simulink model "CopterSim3DEnvironment"  (R2019b)
settings: Solver=ode4  StartTime=0.0  StopTime=inf  FixedStep=0.001  RelTol=1e-3
InitFcn:
  | Init_control;
values from neighbouring files (symbols this model uses):
  Kd_RP_AgngleRate = 0.005    [Init_control.m]    (also in quadFly.sldd)
  Kd_YAW_AngleRate = 0.05    [Init_control.m]    (also in quadFly.sldd)
  Ki_RP_AgngleRate = 0.01    [Init_control.m]    (also in quadFly.sldd)
  Ki_YAW_AngleRate = 0.8    [Init_control.m]    (also in quadFly.sldd)
  Kp_RP_AgngleRate = 0.55    [Init_control.m]    (also in quadFly.sldd)
  Kp_RP_ANGLE = 6.5    [Init_control.m]    (also in quadFly.sldd)
  Kp_YAW_AngleRate = 3.2    [Init_control.m]    (also in quadFly.sldd)
  MAX_CONTROL_ANGLE_RATE_Y = 90    [Init_control.m]    (also in quadFly.sldd = 90.0)
  ModelInit_RPM = 0.0    [quadFly.sldd]
  ModelParam_envAltitude = -41.5260009765625    [quadFly.sldd]
  ModelParam_GlobalNoiseGainSwitch = 1.0    [quadFly.sldd]
  ModelParam_GPSLatLong = 40.1540302 116.2593683    [quadFly.sldd]
  ModelParam_motorCr = 1148.0    [quadFly.sldd]
  ModelParam_motorJm = 0.0001287    [quadFly.sldd]
  ModelParam_motorMinThr = 0.05    [quadFly.sldd]
  ModelParam_motorT = 0.02    [quadFly.sldd]
  ModelParam_motorWb = -141.4    [quadFly.sldd]
  ModelParam_rotorCm = 1.779E-7    [quadFly.sldd]
  ModelParam_rotorCt = 1.105E-5    [quadFly.sldd]
  ModelParam_uavCCm = 0.01 0.01 0.0055    [quadFly.sldd]
  ModelParam_uavCd = 0.073    [quadFly.sldd]
  ModelParam_uavDearo = 0.12    [quadFly.sldd]
  ModelParam_uavJ = 0.0211 0.0 0.0 0.0 0.0219 0.0 0.0 0.0 0.0366    [quadFly.sldd]
  ModelParam_uavMass = 1.4    [quadFly.sldd]
  ModelParam_uavR = 0.225    [quadFly.sldd]
  ModelParam_uavType = 3    [quadFly.sldd]
undefined symbols (not defined in the file or in its folder): DWORK0, DWORK1, DWORK10, DWORK11, DWORK12, DWORK13, DWORK14, DWORK15, DWORK2, DWORK3, DWORK4, DWORK5, DWORK6, DWORK7, DWORK8, DWORK9, earthRadius, KiPitchAttitude, KiRollAttitude, Receive, Send
libraries: simulink x15, ctrl_ADRC_angular_rate x4, aerolibfltsims x3, ctrl_ADRC_TD x2, shared6dof x1, aerolibanimutils x1
(part 3 of 4)

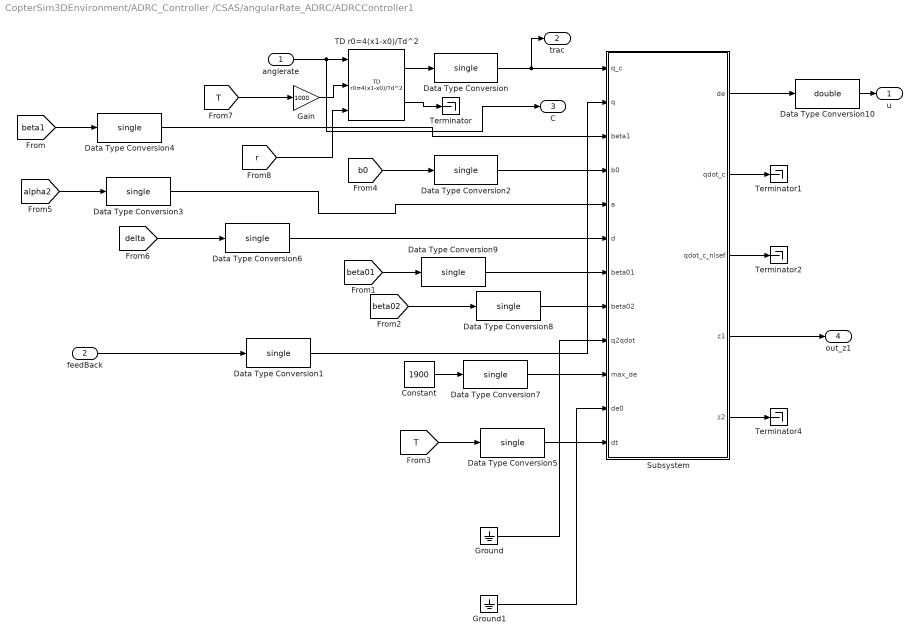
== system CopterSim3DEnvironment/ADRC_Controller /CSAS/angularRate_ADRC/ADRCController1 ==
  anglerate : Inport
  feedBack : Inport  Port=2
  Constant : Constant  Value=1900
  Data Type Conversion{,1..9} (10 alike) : DataTypeConversion  OutDataTypeStr=single
  Data Type Conversion10 : DataTypeConversion  OutDataTypeStr=double
  Gain : Gain  Gain=1000
  Ground : Ground
  Ground1 : Ground
  Subsystem : Subsystem  AncestorBlock=ctrl_ADRC_angular_rate/Subsystem  mask(ADRC angular rate controller){}
      mask help: 二阶ADRC姿态角速率控制
  TD r0=4(x1-x0)/Td^2 : ctrl_ADRC_TD/TD r0=4(x1-x0)//Td^2
  Terminator{,1..2,4} (4 alike) : Terminator
  u : Outport
  trac : Outport  Port=2
  C : Outport  Port=3
  out_z1 : Outport  Port=4
  wires:
  Constant/1 -> Data Type Conversion7/1
  Ground/1 -> Subsystem/9(q2qdot)
  Data Type Conversion1/1 -> Subsystem/2(q)
  Data Type Conversion/1 -> trac/1, Subsystem/1(q_c)
  [beta01] -> Data Type Conversion9/1
  [delta] -> Data Type Conversion6/1
  [r] -> TD r0=4(x1-x0)/Td^2/3
  [beta1] -> Data Type Conversion4/1
  [alpha2] -> Data Type Conversion3/1
  [T] -> Gain/1
  Ground1/1 -> Subsystem/11(de0)
  feedBack/1 -> Data Type Conversion1/1
  [b0] -> Data Type Conversion2/1
  [T] -> Data Type Conversion5/1
  [beta02] -> Data Type Conversion8/1
  Subsystem/5(z2) -> Terminator4/1
  Subsystem/4(z1) -> out_z1/1
  Subsystem/2(qdot_c) -> Terminator1/1
  Subsystem/3(qdot_c_nlsef) -> Terminator2/1
  anglerate/1 -> C/1, TD r0=4(x1-x0)/Td^2/1
  Subsystem/1(de) -> Data Type Conversion10/1
  TD r0=4(x1-x0)/Td^2/2 -> Terminator/1
  TD r0=4(x1-x0)/Td^2/1 -> Data Type Conversion/1
  Data Type Conversion2/1 -> Subsystem/4(b0)
  Data Type Conversion4/1 -> Subsystem/3(beta1)
  Data Type Conversion3/1 -> Subsystem/5(a)
  Data Type Conversion6/1 -> Subsystem/6(d)
  Data Type Conversion5/1 -> Subsystem/12(dt)
  Data Type Conversion7/1 -> Subsystem/10(max_de)
  Data Type Conversion8/1 -> Subsystem/8(beta02)
  Data Type Conversion9/1 -> Subsystem/7(beta01)
  Data Type Conversion10/1 -> u/1
  Gain/1 -> TD r0=4(x1-x0)/Td^2/2

== system CopterSim3DEnvironment/ADRC_Controller /CSAS/angularRate_ADRC/ADRCController2 ==
  anglerate : Inport
  angleRateBack : Inport  Port=2
  Add : Sum  Inputs=+-
  Add1 : Sum  Inputs=+-
  Add2 : Sum  Inputs=+-
  Divide : Product  Inputs=*/
  NLSEF : Subsystem
  TD : Subsystem
  Unit Delay : UnitDelay  SampleTime=-1  HasFrameUpgradeWarning=on
  eso : Subsystem
  u : Outport
  wires:
  anglerate/1 -> TD/1(anglerate)
  TD/1(anglerateV1) -> Add/1
  TD/2(angleAccV2) -> Add1/1
  eso/1(z1) -> Add/2
  eso/2(z2) -> Add1/2
  Add/1 -> NLSEF/1(e1)
  Add1/1 -> NLSEF/2(e2)
  eso/3(z3) -> Add2/2
  NLSEF/1(u0) -> Add2/1
  Add2/1 -> Unit Delay/1, Divide/1
  [b0] -> Divide/2
  Divide/1 -> u/1
  angleRateBack/1 -> eso/1(phi_rate)
  Unit Delay/1 -> eso/2(angle_u)

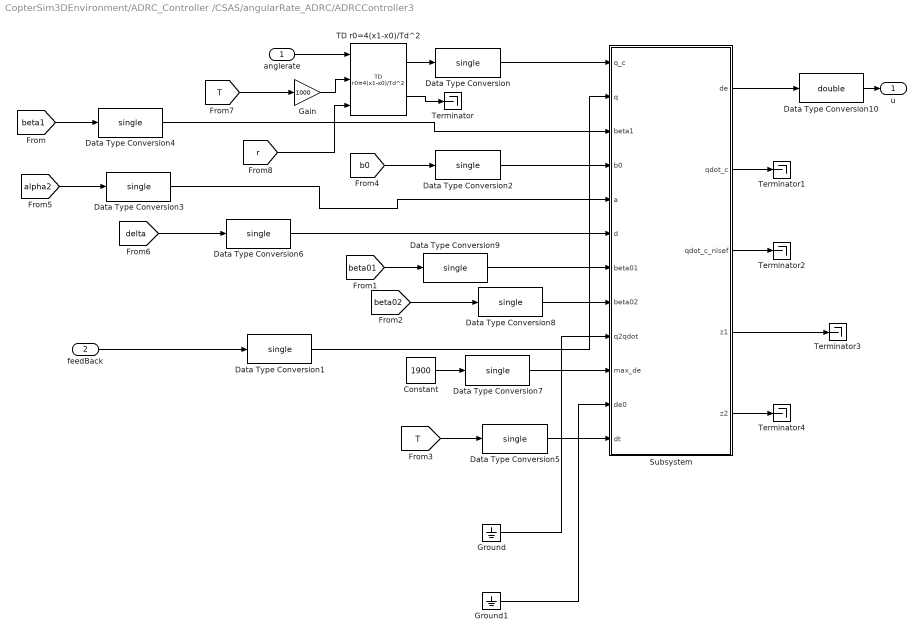
== system CopterSim3DEnvironment/ADRC_Controller /CSAS/angularRate_ADRC/ADRCController3 ==
  anglerate : Inport
  feedBack : Inport  Port=2
  Constant : Constant  Value=1900
  Data Type Conversion{,1..9} (10 alike) : DataTypeConversion  OutDataTypeStr=single
  Data Type Conversion10 : DataTypeConversion  OutDataTypeStr=double
  Gain : Gain  Gain=1000
  Ground : Ground
  Ground1 : Ground
  Subsystem : Subsystem  AncestorBlock=ctrl_ADRC_angular_rate/Subsystem  mask(ADRC angular rate controller){}
      mask help: 二阶ADRC姿态角速率控制
  TD r0=4(x1-x0)/Td^2 : ctrl_ADRC_TD/TD r0=4(x1-x0)//Td^2
  Terminator{,1..4} (5 alike) : Terminator
  u : Outport
  wires:
  Constant/1 -> Data Type Conversion7/1
  Ground/1 -> Subsystem/9(q2qdot)
  Data Type Conversion1/1 -> Subsystem/2(q)
  Data Type Conversion/1 -> Subsystem/1(q_c)
  [beta01] -> Data Type Conversion9/1
  [delta] -> Data Type Conversion6/1
  [r] -> TD r0=4(x1-x0)/Td^2/3
  [beta1] -> Data Type Conversion4/1
  [alpha2] -> Data Type Conversion3/1
  [T] -> Gain/1
  Ground1/1 -> Subsystem/11(de0)
  feedBack/1 -> Data Type Conversion1/1
  [b0] -> Data Type Conversion2/1
  [T] -> Data Type Conversion5/1
  [beta02] -> Data Type Conversion8/1
  Subsystem/5(z2) -> Terminator4/1
  Subsystem/4(z1) -> Terminator3/1
  Subsystem/2(qdot_c) -> Terminator1/1
  Subsystem/3(qdot_c_nlsef) -> Terminator2/1
  anglerate/1 -> TD r0=4(x1-x0)/Td^2/1
  Subsystem/1(de) -> Data Type Conversion10/1
  TD r0=4(x1-x0)/Td^2/2 -> Terminator/1
  TD r0=4(x1-x0)/Td^2/1 -> Data Type Conversion/1
  Data Type Conversion2/1 -> Subsystem/4(b0)
  Data Type Conversion4/1 -> Subsystem/3(beta1)
  Data Type Conversion3/1 -> Subsystem/5(a)
  Data Type Conversion6/1 -> Subsystem/6(d)
  Data Type Conversion5/1 -> Subsystem/12(dt)
  Data Type Conversion7/1 -> Subsystem/10(max_de)
  Data Type Conversion8/1 -> Subsystem/8(beta02)
  Data Type Conversion9/1 -> Subsystem/7(beta01)
  Data Type Conversion10/1 -> u/1
  Gain/1 -> TD r0=4(x1-x0)/Td^2/2

== system CopterSim3DEnvironment/ADRC_Controller /CSAS/angularRate_ADRC/Subsystem ==
  yaw : Inport
  q : Inport  Port=2
  r : Inport  Port=3
  pitchRateCom : Inport  Port=4
  Sum17 : Sum  Inputs=|-+
  Sum21 : Sum  Inputs=|-+
  pitch_rate : simulink/Continuous/PID Controller  Controller=PID  Form=Parallel  TimeDomain=Discrete-time  SampleTime=-1  IntegratorMethod=Forward Euler  FilterMethod=Forward Euler  ControllerParametersSource=internal  P=Kp_RP_AgngleRate  I=Ki_RP_AgngleRate  D=Kd_RP_AgngleRate  UseFilter=off  N=100  TunerSelectOption=Transfer Function Based (PID Tuner App)  InitialConditionSource=internal  InitialConditionForIntegrator=0  InitialConditionForFilter=0  DifferentiatorICPrevScaledInput=0  ExternalReset=none  TrackingMode=off  Kt=1  LimitOutput=on  UpperSaturationLimit=500  LowerSaturationLimit=-500  LinearizeAsGain=on  AntiWindupMode=back-calculation  Kb=1  POutMin=[]  POutMax=[]  IOutMin=[]  IOutMax=[]  DOutMin=[]  DOutMax=[]  NOutMin=[]  NOutMax=[]  SumOutMin=[]  SumOutMax=[]  SaturationOutMin=[]  SaturationOutMax=[]  PParamMin=[]  PParamMax=[]  IParamMin=[]  IParamMax=[]  DParamMin=[]  DParamMax=[]  NParamMin=[]  NParamMax=[]  KbParamMin=[]  KbParamMax=[]  KtParamMin=[]  KtParamMax=[]  KbOutMin=[]  KbOutMax=[]  KtOutMin=[]  KtOutMax=[]  IntegratorOutMin=[]  IntegratorOutMax=[]  FilterOutMin=[]  FilterOutMax=[]  SumI1OutMin=[]  SumI1OutMax=[]  SumI2OutMin=[]  SumI2OutMax=[]  SumI3OutMin=[]  SumI3OutMax=[]  SumI4OutMin=[]  SumI4OutMax=[]  SumDOutMin=[]  SumDOutMax=[]  DifferentiatorOutMin=[]  DifferentiatorOutMax=[]  FilterDiffOutCoefMin=[]  FilterDiffOutCoefMax=[]  ReciprocalOutMin=[]  ReciprocalOutMax=[]  SumDenOutMin=[]  SumDenOutMax=[]  SumNumOutMin=[]  SumNumOutMax=[]  DivideOutMin=[]  DivideOutMax=[]  IntegratorContinuousStateAttributes=''  IntegratorStateMustResolveToSignalObject=off  IntegratorRTWStateStorageClass=Auto  FilterContinuousStateAttributes=''  FilterStateMustResolveToSignalObject=off  FilterRTWStateStorageClass=Auto  ParallelPVariant=InternalParameters  IdealPVariant=Disabled  IVariant=InternalParameters  DVariant=InternalParameters  IntegratorVariant=Discrete  SatVariant=Enabled  AWVariant=BackCalculation  PCopyVariant=Disabled  TRVariant=Disabled  FdbkBlocksVariant=Forward  IdealPFdbkVariant=Disabled  SatFdbkVariant=Disabled  DerivativeFilterVariant=Differentiator  NVariant=Passthrough  NCopyVariant=Disabled_SignalSpec  FilterICVariant=InternalICsDifferentiator  IntegratorICVariant=InternalICs  ExternalResetVariant=Disabled  TRSumVariant=Passthrough  SumFdbkVariant=Disabled  SumVariant=Sum_PID
  yaw_rate : simulink/Continuous/PID Controller  Controller=PID  Form=Parallel  TimeDomain=Discrete-time  SampleTime=-1  IntegratorMethod=Forward Euler  FilterMethod=Forward Euler  ControllerParametersSource=internal  P=Kp_YAW_AngleRate  I=Ki_YAW_AngleRate  D=Kd_YAW_AngleRate  UseFilter=off  N=100  TunerSelectOption=Transfer Function Based (PID Tuner App)  InitialConditionSource=internal  InitialConditionForIntegrator=0  InitialConditionForFilter=0  DifferentiatorICPrevScaledInput=0  ExternalReset=none  TrackingMode=off  Kt=1  LimitOutput=on  UpperSaturationLimit=500  LowerSaturationLimit=-500  LinearizeAsGain=on  AntiWindupMode=back-calculation  Kb=1  POutMin=[]  POutMax=[]  IOutMin=[]  IOutMax=[]  DOutMin=[]  DOutMax=[]  NOutMin=[]  NOutMax=[]  SumOutMin=[]  SumOutMax=[]  SaturationOutMin=[]  SaturationOutMax=[]  PParamMin=[]  PParamMax=[]  IParamMin=[]  IParamMax=[]  DParamMin=[]  DParamMax=[]  NParamMin=[]  NParamMax=[]  KbParamMin=[]  KbParamMax=[]  KtParamMin=[]  KtParamMax=[]  KbOutMin=[]  KbOutMax=[]  KtOutMin=[]  KtOutMax=[]  IntegratorOutMin=[]  IntegratorOutMax=[]  FilterOutMin=[]  FilterOutMax=[]  SumI1OutMin=[]  SumI1OutMax=[]  SumI2OutMin=[]  SumI2OutMax=[]  SumI3OutMin=[]  SumI3OutMax=[]  SumI4OutMin=[]  SumI4OutMax=[]  SumDOutMin=[]  SumDOutMax=[]  DifferentiatorOutMin=[]  DifferentiatorOutMax=[]  FilterDiffOutCoefMin=[]  FilterDiffOutCoefMax=[]  ReciprocalOutMin=[]  ReciprocalOutMax=[]  SumDenOutMin=[]  SumDenOutMax=[]  SumNumOutMin=[]  SumNumOutMax=[]  DivideOutMin=[]  DivideOutMax=[]  IntegratorContinuousStateAttributes=''  IntegratorStateMustResolveToSignalObject=off  IntegratorRTWStateStorageClass=Auto  FilterContinuousStateAttributes=''  FilterStateMustResolveToSignalObject=off  FilterRTWStateStorageClass=Auto  ParallelPVariant=InternalParameters  IdealPVariant=Disabled  IVariant=InternalParameters  DVariant=InternalParameters  IntegratorVariant=Discrete  SatVariant=Enabled  AWVariant=BackCalculation  PCopyVariant=Disabled  TRVariant=Disabled  FdbkBlocksVariant=Forward  IdealPFdbkVariant=Disabled  SatFdbkVariant=Disabled  DerivativeFilterVariant=Differentiator  NVariant=Passthrough  NCopyVariant=Disabled_SignalSpec  FilterICVariant=InternalICsDifferentiator  IntegratorICVariant=InternalICs  ExternalResetVariant=Disabled  TRSumVariant=Passthrough  SumFdbkVariant=Disabled  SumVariant=Sum_PID
  Pitch : Outport  VectorParamsAs1DForOutWhenUnconnected=off
  Yaw : Outport  Port=2  VectorParamsAs1DForOutWhenUnconnected=off
  wires:
  Sum17/1 -> yaw_rate/1
  Sum21/1 -> pitch_rate/1
  q/1 -> Sum21/1
  yaw_rate/1 -> Yaw/1
  pitch_rate/1 -> Pitch/1
  r/1 -> Sum17/1
  yaw/1 -> Sum17/2
  pitchRateCom/1 -> Sum21/2

== system CopterSim3DEnvironment/ADRC_Controller /CSAS/angularRate_ADRC/ADRCController1/Subsystem ==
  q_c : Inport
  q : Inport  Port=2
  beta1 : Inport  Port=3
  b0 : Inport  Port=4
  a : Inport  Port=5
  d : Inport  Port=6
  beta01 : Inport  Port=7
  beta02 : Inport  Port=8
  q2qdot : Inport  Port=9
  max_de : Inport  Port=10
  de0 : Inport  Port=11
  dt : Inport  Port=12
  Divide : Product  Inputs=*/
  Gain : Gain  Gain=-1
  Product : Product
  Saturation Dynamic : simulink/Discontinuities/Saturation Dynamic  OutMin=[]  OutMax=[]  OutDataTypeStr=Inherit: Same as second input  OutDataType=fixdt(1, 16)  OutScaling=2^-10  DoSatur=off
  Sum : Sum  Inputs=|+-
  Terminator : Terminator
  Terminator1 : Terminator
  alpha : Constant  Value=0.5  OutDataTypeStr=single
  b1 : InportShadow  Port=4
  delta : Constant  Value=200  OutDataTypeStr=single
  eso : Subsystem  mask(eso){}
      mask help: 二阶带模型信息的扩张状态观测器
  max_de1 : InportShadow  Port=10
  nlsef : Subsystem  mask(nlsef){}
      mask help: 非线性误差反馈控制律
  de : Outport  VectorParamsAs1DForOutWhenUnconnected=off
  qdot_c : Outport  Port=2  VectorParamsAs1DForOutWhenUnconnected=off
  qdot_c_nlsef : Outport  Port=3  VectorParamsAs1DForOutWhenUnconnected=off
  z1 : Outport  Port=4  VectorParamsAs1DForOutWhenUnconnected=off
  z2 : Outport  Port=5  VectorParamsAs1DForOutWhenUnconnected=off
  wires:
  q/1 -> eso/2(y)
  Product/1 -> Terminator1/1
  b1/1 -> eso/3(b0)
  max_de1/1 -> eso/4(max_de)
  de0/1 -> eso/5(de0)
  q2qdot/1 -> eso/11(Mq), Product/2
  dt/1 -> eso/10(dt)
  beta02/1 -> eso/9(beta02)
  beta01/1 -> eso/8(beta01)
  d/1 -> eso/7(d)
  a/1 -> eso/6(a)
  eso/1(z2) -> Sum/2, z2/1
  eso/2(z1) -> nlsef/5(z1), z1/1, Product/1
  Saturation Dynamic/1 -> Terminator/1, eso/1(u)
  Gain/1 -> Saturation Dynamic/3
  max_de/1 -> Gain/1, Saturation Dynamic/1
  Divide/1 -> de/1, Saturation Dynamic/2
  b0/1 -> Divide/2
  Sum/1 -> Divide/1, qdot_c/1
  nlsef/1(u0) -> Sum/1, qdot_c_nlsef/1
  beta1/1 -> nlsef/4(beta1)
  q_c/1 -> nlsef/1(v)
  delta/1 -> nlsef/3(d)
  alpha/1 -> nlsef/2(a)

== system CopterSim3DEnvironment/ADRC_Controller /CSAS/angularRate_ADRC/ADRCController2/NLSEF ==
  e1 : Inport
  e2 : Inport  Port=2
  Add : Sum
  Product : Product
  Product1 : Product
  Subsystem : Subsystem
  Subsystem1 : Subsystem
  u0 : Outport
  wires:
  e1/1 -> Subsystem/1(e)
  e2/1 -> Subsystem1/1(e)
  Subsystem/1(fal) -> Product/2
  Subsystem1/1(fal) -> Product1/2
  [alpha01] -> Subsystem/2(a)
  [delta0] -> Subsystem1/3(d), Subsystem/3(d)
  [alpha02] -> Subsystem1/2(a)
  [beta01] -> Product/1
  [beta02] -> Product1/1
  Product/1 -> Add/1
  Product1/1 -> Add/2
  Add/1 -> u0/1

== system CopterSim3DEnvironment/ADRC_Controller /CSAS/angularRate_ADRC/ADRCController2/TD ==
  anglerate : Inport
  Add : Sum
  Add1 : Sum
  Product : Product
  Product1 : Product
  Unit Delay : UnitDelay  SampleTime=-1  HasFrameUpgradeWarning=on
  Unit Delay1 : UnitDelay  SampleTime=-1  HasFrameUpgradeWarning=on
  Unit Delay2 : UnitDelay  SampleTime=-1  HasFrameUpgradeWarning=on
  fhan : Subsystem
  anglerateV1 : Outport
  angleAccV2 : Outport  Port=2
  wires:
  anglerate/1 -> fhan/1(rollrate)
  Unit Delay2/1 -> Product/1, fhan/3(v2)
  [T] -> Product1/2, Product/2
  Product/1 -> Add/1
  Add/1 -> Unit Delay/1, fhan/2(v1), anglerateV1/1
  fhan/1(fhan) -> Product1/1
  Product1/1 -> Add1/1
  Add1/1 -> Unit Delay1/1, Unit Delay2/1, angleAccV2/1
  Unit Delay/1 -> Add/2
  Unit Delay1/1 -> Add1/2

== system CopterSim3DEnvironment/ADRC_Controller /CSAS/angularRate_ADRC/ADRCController2/eso ==
  phi_rate : Inport
  angle_u : Inport  Port=2
  Add : Sum  Inputs=-+
  Add1 : Sum  Inputs=-+
  Add2 : Sum
  Add3 : Sum  Inputs=-++
  Add4 : Sum
  Add5 : Sum
  Product{1..4,6} (5 alike) : Product
  Product5 : Product  Inputs=3
  Subsystem : Subsystem
  Subsystem1 : Subsystem
  Unit Delay{,1..3} (4 alike) : UnitDelay  SampleTime=-1  HasFrameUpgradeWarning=on
  z1 : Outport
  z2 : Outport  Port=2
  z3 : Outport  Port=3
  wires:
  phi_rate/1 -> Add/1
  Add/1 -> Subsystem1/1(e), Subsystem/1(e), Product6/1
  [beta1] -> Product6/2
  Product6/1 -> Add1/1
  Add1/1 -> Product1/1
  [T] -> Product5/3, Product4/1, Product1/2
  Product1/1 -> Add2/1
  Add2/1 -> Unit Delay/1, Unit Delay2/1, z1/1
  [delta] -> Subsystem1/3(d), Subsystem/3(d)
  [alpha1] -> Subsystem/2(a)
  [beta2] -> Product2/2
  Subsystem/1(fal) -> Product2/1
  Product2/1 -> Add3/1
  angle_u/1 -> Product3/1
  [b0] -> Product3/2
  Product3/1 -> Add3/2
  Add3/1 -> Product4/2
  Add4/1 -> Unit Delay1/1, Add1/2, z2/1
  Product4/1 -> Add4/1
  Add5/1 -> Unit Delay3/1, Add3/3, z3/1
  [beta3] -> Product5/1
  Product5/1 -> Add5/1
  Subsystem1/1(fal) -> Product5/2
  [alpha2] -> Subsystem1/2(a)
  Unit Delay/1 -> Add/2
  Unit Delay1/1 -> Add4/2
  Unit Delay2/1 -> Add2/2
  Unit Delay3/1 -> Add5/2

== system CopterSim3DEnvironment/ADRC_Controller /CSAS/angularRate_ADRC/ADRCController3/Subsystem ==
  q_c : Inport
  q : Inport  Port=2
  beta1 : Inport  Port=3
  b0 : Inport  Port=4
  a : Inport  Port=5
  d : Inport  Port=6
  beta01 : Inport  Port=7
  beta02 : Inport  Port=8
  q2qdot : Inport  Port=9
  max_de : Inport  Port=10
  de0 : Inport  Port=11
  dt : Inport  Port=12
  Divide : Product  Inputs=*/
  Gain : Gain  Gain=-1
  Product : Product
  Saturation Dynamic : simulink/Discontinuities/Saturation Dynamic  OutMin=[]  OutMax=[]  OutDataTypeStr=Inherit: Same as second input  OutDataType=fixdt(1, 16)  OutScaling=2^-10  DoSatur=off
  Sum : Sum  Inputs=|+-
  Terminator : Terminator
  Terminator1 : Terminator
  alpha : Constant  Value=0.5  OutDataTypeStr=single
  b1 : InportShadow  Port=4
  delta : Constant  Value=200  OutDataTypeStr=single
  eso : Subsystem  mask(eso){}
      mask help: 二阶带模型信息的扩张状态观测器
  max_de1 : InportShadow  Port=10
  nlsef : Subsystem  mask(nlsef){}
      mask help: 非线性误差反馈控制律
  de : Outport  VectorParamsAs1DForOutWhenUnconnected=off
  qdot_c : Outport  Port=2  VectorParamsAs1DForOutWhenUnconnected=off
  qdot_c_nlsef : Outport  Port=3  VectorParamsAs1DForOutWhenUnconnected=off
  z1 : Outport  Port=4  VectorParamsAs1DForOutWhenUnconnected=off
  z2 : Outport  Port=5  VectorParamsAs1DForOutWhenUnconnected=off
  wires:
  q/1 -> eso/2(y)
  Product/1 -> Terminator1/1
  b1/1 -> eso/3(b0)
  max_de1/1 -> eso/4(max_de)
  de0/1 -> eso/5(de0)
  q2qdot/1 -> eso/11(Mq), Product/2
  dt/1 -> eso/10(dt)
  beta02/1 -> eso/9(beta02)
  beta01/1 -> eso/8(beta01)
  d/1 -> eso/7(d)
  a/1 -> eso/6(a)
  eso/1(z2) -> Sum/2, z2/1
  eso/2(z1) -> nlsef/5(z1), z1/1, Product/1
  Saturation Dynamic/1 -> Terminator/1, eso/1(u)
  Gain/1 -> Saturation Dynamic/3
  max_de/1 -> Gain/1, Saturation Dynamic/1
  Divide/1 -> de/1, Saturation Dynamic/2
  b0/1 -> Divide/2
  Sum/1 -> Divide/1, qdot_c/1
  nlsef/1(u0) -> Sum/1, qdot_c_nlsef/1
  beta1/1 -> nlsef/4(beta1)
  q_c/1 -> nlsef/1(v)
  delta/1 -> nlsef/3(d)
  alpha/1 -> nlsef/2(a)

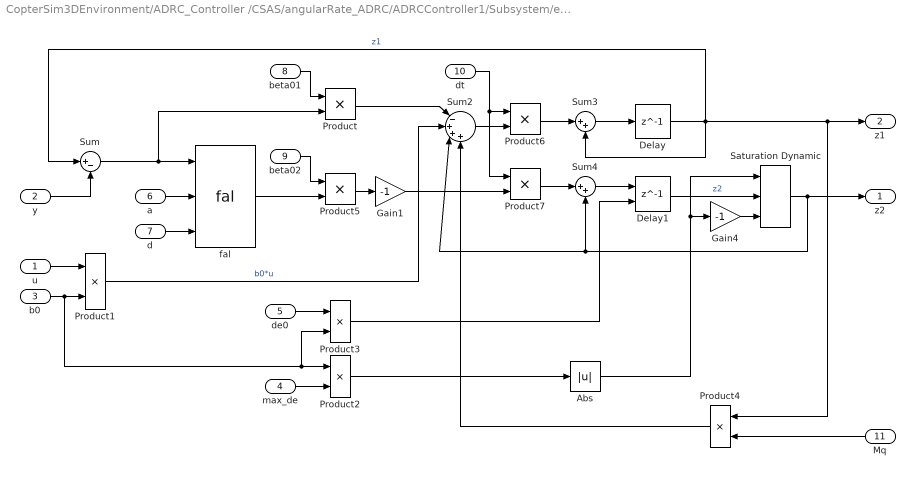
== system CopterSim3DEnvironment/ADRC_Controller /CSAS/angularRate_ADRC/ADRCController1/Subsystem/eso ==
  u : Inport
  y : Inport  Port=2
  b0 : Inport  Port=3
  max_de : Inport  Port=4
  de0 : Inport  Port=5
  a : Inport  Port=6
  d : Inport  Port=7
  beta01 : Inport  Port=8
  beta02 : Inport  Port=9
  dt : Inport  Port=10
  Mq : Inport  Port=11
  Abs : Abs
  Delay : Delay  DelayLength=1
  Delay1 : Delay  DelayLength=1  InitialConditionSource=Input port
      settings: InputPortMap=u0,p4
  Gain1 : Gain  Gain=-1
      settings: AttributesFormatString=%<Gain>
  Gain4 : Gain  Gain=-1
  Product{,1..7} (8 alike) : Product
  Saturation Dynamic : simulink/Discontinuities/Saturation Dynamic  OutMin=[]  OutMax=[]  OutDataTypeStr=Inherit: Same as second input  OutDataType=fixdt(1, 16)  OutScaling=2^-10  DoSatur=off
  Sum : Sum  Inputs=|+-
  Sum2 : Sum  Inputs=|-+++
  Sum3 : Sum  Inputs=|++
  Sum4 : Sum  Inputs=|++
  fal : ctrl_ADRC_angular_rate/Subsystem/nlsef/fal
  z2 : Outport  VectorParamsAs1DForOutWhenUnconnected=off
  z1 : Outport  Port=2  VectorParamsAs1DForOutWhenUnconnected=off
  wires:
  Gain4/1 -> Saturation Dynamic/3
  dt/1 -> Product7/1, Product6/1
  Product5/1 -> Gain1/1
  fal/1 -> Product5/2
  beta02/1 -> Product5/1
  beta01/1 -> Product/1
  Product7/1 -> Sum4/1
  Sum4/1 -> Delay1/1
  Product1/1 -> Sum2/2  "b0*u"
  Delay1/1 -> Saturation Dynamic/2  "z2"
  a/1 -> fal/2
  Sum/1 -> fal/1, Product/2
  d/1 -> fal/3
  max_de/1 -> Product2/2
  u/1 -> Product1/1
  Delay/1 -> Sum/1, z1/1, Product4/1, Sum3/2  "z1"
  Mq/1 -> Product4/2
  Gain1/1 -> Product7/2
  b0/1 -> Product3/2, Product2/1, Product1/2
  Product4/1 -> Sum2/4
  y/1 -> Sum/2
  Product6/1 -> Sum3/1
  Saturation Dynamic/1 -> Sum4/2, Sum2/3, z2/1
  Product3/1 -> Delay1/2
  Product2/1 -> Abs/1
  Product/1 -> Sum2/1
  Sum3/1 -> Delay/1
  Sum2/1 -> Product6/2
  de0/1 -> Product3/1
  Abs/1 -> Gain4/1, Saturation Dynamic/1

== system CopterSim3DEnvironment/ADRC_Controller /CSAS/angularRate_ADRC/ADRCController1/Subsystem/nlsef ==
  v : Inport
  a : Inport  Port=2
  d : Inport  Port=3
  beta1 : Inport  Port=4
  z1 : Inport  Port=5
  Product : Product
  Sum : Sum  Inputs=|+-
  fal : Subsystem  mask(fal){}
      mask help: 最速综合控制函数
  u0 : Outport  VectorParamsAs1DForOutWhenUnconnected=off
  wires:
  Product/1 -> u0/1
  beta1/1 -> Product/2
  fal/1(fal) -> Product/1
  d/1 -> fal/3(d)
  a/1 -> fal/2(a)
  Sum/1 -> fal/1(e)
  v/1 -> Sum/1
  z1/1 -> Sum/2

== system CopterSim3DEnvironment/ADRC_Controller /CSAS/angularRate_ADRC/ADRCController2/NLSEF/Subsystem ==
  e : Inport
  a : Inport  Port=2
  d : Inport  Port=3
  Abs : Abs
  Constant1 : Constant  OutDataTypeStr=single
  Divide : Product  Inputs=*/
  If : If
  If Action Subsystem1 : Subsystem  TreatAsAtomicUnit=on
  If Action Subsystem3 : Subsystem  TreatAsAtomicUnit=on
  Merge : Merge
  Product : Product
  Product1 : Product
  Sign : Signum
  Sum : Sum  Inputs=+-
  Sum1 : Sum  Inputs=|+-
  pow : Math  Operator=pow  SaturateOnIntegerOverflow=on
  pow1 : Math  Operator=pow  SaturateOnIntegerOverflow=on
  fal : Outport  VectorParamsAs1DForOutWhenUnconnected=off
  wires:
  Constant1/1 -> Sum/1, Product1/2
  Sum1/1 -> If/1  "|x|-d"
  Sign/1 -> Product/1  "sign(x)"
  pow1/1 -> Divide/2  "d^(1-a)"
  Sum/1 -> pow1/2
  If Action Subsystem3/1(Out1) -> Merge/1
  Merge/1 -> fal/1
  pow/1 -> Product/2  "|x|^a"
  Product1/1 -> Sum1/2, pow1/1  "d"
  d/1 -> Product1/1
  If/2 -> If Action Subsystem1/Action  "|x|<=d"
  Abs/1 -> Sum1/1, pow/1  "|x|"
  Product/1 -> If Action Subsystem3/1(In1)  "sign(x)|x|^a"
  e/1 -> Abs/1, Divide/1, Sign/1  "x"
  If/1 -> If Action Subsystem3/Action  "|x|>d"
  Divide/1 -> If Action Subsystem1/1(In1)
  If Action Subsystem1/1(Out1) -> Merge/2
  a/1 -> pow/2, Sum/2  "a"

== system CopterSim3DEnvironment/ADRC_Controller /CSAS/angularRate_ADRC/ADRCController2/NLSEF/Subsystem1 ==
  e : Inport
  a : Inport  Port=2
  d : Inport  Port=3
  Abs : Abs
  Constant1 : Constant  OutDataTypeStr=single
  Divide : Product  Inputs=*/
  If : If
  If Action Subsystem1 : Subsystem  TreatAsAtomicUnit=on
  If Action Subsystem3 : Subsystem  TreatAsAtomicUnit=on
  Merge : Merge
  Product : Product
  Product1 : Product
  Sign : Signum
  Sum : Sum  Inputs=+-
  Sum1 : Sum  Inputs=|+-
  pow : Math  Operator=pow  SaturateOnIntegerOverflow=on
  pow1 : Math  Operator=pow  SaturateOnIntegerOverflow=on
  fal : Outport  VectorParamsAs1DForOutWhenUnconnected=off
  wires:
  Constant1/1 -> Sum/1, Product1/2
  Sum1/1 -> If/1  "|x|-d"
  Sign/1 -> Product/1  "sign(x)"
  pow1/1 -> Divide/2  "d^(1-a)"
  Sum/1 -> pow1/2
  If Action Subsystem3/1(Out1) -> Merge/1
  Merge/1 -> fal/1
  pow/1 -> Product/2  "|x|^a"
  Product1/1 -> Sum1/2, pow1/1  "d"
  d/1 -> Product1/1
  If/2 -> If Action Subsystem1/Action  "|x|<=d"
  Abs/1 -> Sum1/1, pow/1  "|x|"
  Product/1 -> If Action Subsystem3/1(In1)  "sign(x)|x|^a"
  e/1 -> Abs/1, Divide/1, Sign/1  "x"
  If/1 -> If Action Subsystem3/Action  "|x|>d"
  Divide/1 -> If Action Subsystem1/1(In1)
  If Action Subsystem1/1(Out1) -> Merge/2
  a/1 -> pow/2, Sum/2  "a"

== system CopterSim3DEnvironment/ADRC_Controller /CSAS/angularRate_ADRC/ADRCController2/TD/fhan ==
  rollrate : Inport
  v1 : Inport  Port=2
  v2 : Inport  Port=3
  Add : Sum  Inputs=-+
  Constant : Constant  Value=-1
  Fhan : Subsystem
  Product : Product
  a : Subsystem
  a0 : Subsystem
  d : Subsystem
  d0 : Subsystem
  y : Subsystem
  fhan : Outport
  wires:
  rollrate/1 -> Add/1
  v1/1 -> Add/2
  [r] -> a0/2(r), Fhan/3(r), d/1(r)
  [h] -> y/3(h), a/6(h), d0/2(h), d/2(h)
  d/1(d) -> a/3(d), a0/1(d), Fhan/2(d), d0/1(d)
  Add/1 -> y/1(e)
  v2/1 -> a/1(v2), y/2(v2)
  a/1(a) -> Fhan/1(a)
  Fhan/1(Out1) -> Product/1
  y/1(y) -> a/4(y), a0/3(y)
  a0/1(a0) -> a/2(a0)
  d0/1(d0) -> a/5(d0)
  Constant/1 -> Product/2
  Product/1 -> fhan/1

== system CopterSim3DEnvironment/ADRC_Controller /CSAS/angularRate_ADRC/ADRCController2/eso/Subsystem ==
  e : Inport
  a : Inport  Port=2
  d : Inport  Port=3
  Abs : Abs
  Constant1 : Constant  OutDataTypeStr=single
  Divide : Product  Inputs=*/
  If : If
  If Action Subsystem1 : Subsystem  TreatAsAtomicUnit=on
  If Action Subsystem3 : Subsystem  TreatAsAtomicUnit=on
  Merge : Merge
  Product : Product
  Product1 : Product
  Sign : Signum
  Sum : Sum  Inputs=+-
  Sum1 : Sum  Inputs=|+-
  pow : Math  Operator=pow  SaturateOnIntegerOverflow=on
  pow1 : Math  Operator=pow  SaturateOnIntegerOverflow=on
  fal : Outport  VectorParamsAs1DForOutWhenUnconnected=off
  wires:
  Constant1/1 -> Sum/1, Product1/2
  Sum1/1 -> If/1  "|x|-d"
  Sign/1 -> Product/1  "sign(x)"
  pow1/1 -> Divide/2  "d^(1-a)"
  Sum/1 -> pow1/2
  If Action Subsystem3/1(Out1) -> Merge/1
  Merge/1 -> fal/1
  pow/1 -> Product/2  "|x|^a"
  Product1/1 -> Sum1/2, pow1/1  "d"
  d/1 -> Product1/1
  If/2 -> If Action Subsystem1/Action  "|x|<=d"
  Abs/1 -> Sum1/1, pow/1  "|x|"
  Product/1 -> If Action Subsystem3/1(In1)  "sign(x)|x|^a"
  e/1 -> Abs/1, Divide/1, Sign/1  "x"
  If/1 -> If Action Subsystem3/Action  "|x|>d"
  Divide/1 -> If Action Subsystem1/1(In1)
  If Action Subsystem1/1(Out1) -> Merge/2
  a/1 -> pow/2, Sum/2  "a"

== system CopterSim3DEnvironment/ADRC_Controller /CSAS/angularRate_ADRC/ADRCController2/eso/Subsystem1 ==
  e : Inport
  a : Inport  Port=2
  d : Inport  Port=3
  Abs : Abs
  Constant1 : Constant  OutDataTypeStr=single
  Divide : Product  Inputs=*/
  If : If
  If Action Subsystem : Subsystem  TreatAsAtomicUnit=on
  If Action Subsystem1 : Subsystem  TreatAsAtomicUnit=on
  Merge : Merge
  Product : Product
  Product1 : Product
  Sign : Signum
  Sum : Sum  Inputs=+-
  Sum1 : Sum  Inputs=|+-
  pow : Math  Operator=pow  SaturateOnIntegerOverflow=on
  pow1 : Math  Operator=pow  SaturateOnIntegerOverflow=on
  fal : Outport  VectorParamsAs1DForOutWhenUnconnected=off
  wires:
  Constant1/1 -> Sum/1, Product1/2
  Sum1/1 -> If/1  "|x|-d"
  Sign/1 -> Product/1  "sign(x)"
  pow1/1 -> Divide/2  "d^(1-a)"
  Sum/1 -> pow1/2
  If Action Subsystem1/1(Out1) -> Merge/1
  Merge/1 -> fal/1
  pow/1 -> Product/2  "|x|^a"
  Product1/1 -> Sum1/2, pow1/1  "d"
  d/1 -> Product1/1
  If/2 -> If Action Subsystem/Action  "|x|<=d"
  Abs/1 -> Sum1/1, pow/1  "|x|"
  Product/1 -> If Action Subsystem1/1(In1)  "sign(x)|x|^a"
  e/1 -> Abs/1, Divide/1, Sign/1  "x"
  If/1 -> If Action Subsystem1/Action  "|x|>d"
  Divide/1 -> If Action Subsystem/1(In1)
  If Action Subsystem/1(Out1) -> Merge/2
  a/1 -> pow/2, Sum/2  "a"

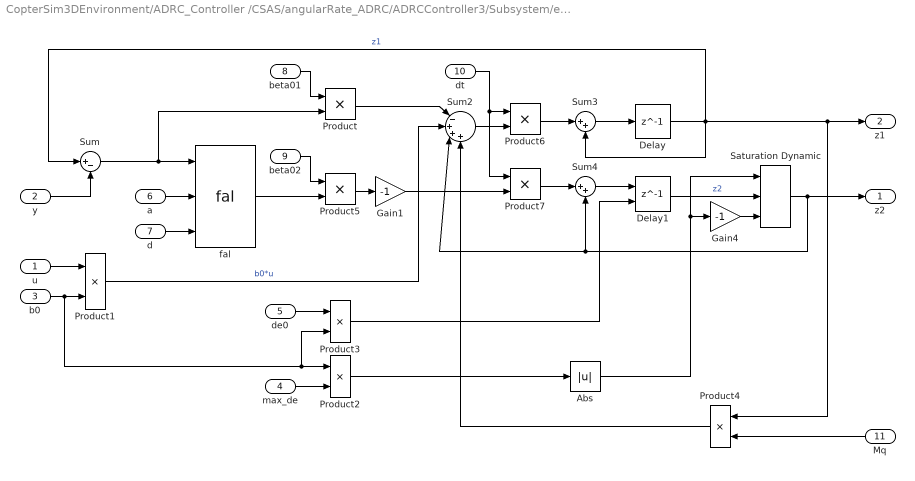
== system CopterSim3DEnvironment/ADRC_Controller /CSAS/angularRate_ADRC/ADRCController3/Subsystem/eso ==
  u : Inport
  y : Inport  Port=2
  b0 : Inport  Port=3
  max_de : Inport  Port=4
  de0 : Inport  Port=5
  a : Inport  Port=6
  d : Inport  Port=7
  beta01 : Inport  Port=8
  beta02 : Inport  Port=9
  dt : Inport  Port=10
  Mq : Inport  Port=11
  Abs : Abs
  Delay : Delay  DelayLength=1
  Delay1 : Delay  DelayLength=1  InitialConditionSource=Input port
      settings: InputPortMap=u0,p4
  Gain1 : Gain  Gain=-1
      settings: AttributesFormatString=%<Gain>
  Gain4 : Gain  Gain=-1
  Product{,1..7} (8 alike) : Product
  Saturation Dynamic : simulink/Discontinuities/Saturation Dynamic  OutMin=[]  OutMax=[]  OutDataTypeStr=Inherit: Same as second input  OutDataType=fixdt(1, 16)  OutScaling=2^-10  DoSatur=off
  Sum : Sum  Inputs=|+-
  Sum2 : Sum  Inputs=|-+++
  Sum3 : Sum  Inputs=|++
  Sum4 : Sum  Inputs=|++
  fal : ctrl_ADRC_angular_rate/Subsystem/nlsef/fal
  z2 : Outport  VectorParamsAs1DForOutWhenUnconnected=off
  z1 : Outport  Port=2  VectorParamsAs1DForOutWhenUnconnected=off
  wires:
  Gain4/1 -> Saturation Dynamic/3
  dt/1 -> Product7/1, Product6/1
  Product5/1 -> Gain1/1
  fal/1 -> Product5/2
  beta02/1 -> Product5/1
  beta01/1 -> Product/1
  Product7/1 -> Sum4/1
  Sum4/1 -> Delay1/1
  Product1/1 -> Sum2/2  "b0*u"
  Delay1/1 -> Saturation Dynamic/2  "z2"
  a/1 -> fal/2
  Sum/1 -> fal/1, Product/2
  d/1 -> fal/3
  max_de/1 -> Product2/2
  u/1 -> Product1/1
  Delay/1 -> Sum/1, z1/1, Product4/1, Sum3/2  "z1"
  Mq/1 -> Product4/2
  Gain1/1 -> Product7/2
  b0/1 -> Product3/2, Product2/1, Product1/2
  Product4/1 -> Sum2/4
  y/1 -> Sum/2
  Product6/1 -> Sum3/1
  Saturation Dynamic/1 -> Sum4/2, Sum2/3, z2/1
  Product3/1 -> Delay1/2
  Product2/1 -> Abs/1
  Product/1 -> Sum2/1
  Sum3/1 -> Delay/1
  Sum2/1 -> Product6/2
  de0/1 -> Product3/1
  Abs/1 -> Gain4/1, Saturation Dynamic/1

== system CopterSim3DEnvironment/ADRC_Controller /CSAS/angularRate_ADRC/ADRCController3/Subsystem/nlsef ==
  v : Inport
  a : Inport  Port=2
  d : Inport  Port=3
  beta1 : Inport  Port=4
  z1 : Inport  Port=5
  Product : Product
  Sum : Sum  Inputs=|+-
  fal : Subsystem  mask(fal){}
      mask help: 最速综合控制函数
  u0 : Outport  VectorParamsAs1DForOutWhenUnconnected=off
  wires:
  Product/1 -> u0/1
  beta1/1 -> Product/2
  fal/1(fal) -> Product/1
  d/1 -> fal/3(d)
  a/1 -> fal/2(a)
  Sum/1 -> fal/1(e)
  v/1 -> Sum/1
  z1/1 -> Sum/2

== system CopterSim3DEnvironment/ADRC_Controller /CSAS/angularRate_ADRC/ADRCController1/Subsystem/nlsef/fal ==
  e : Inport
  a : Inport  Port=2
  d : Inport  Port=3
  Abs : Abs
  Constant1 : Constant  OutDataTypeStr=single
  Divide : Product  Inputs=*/
  If : If
  If Action Subsystem : Subsystem  TreatAsAtomicUnit=on
  If Action Subsystem2 : ctrl_ADRC_angular_rate/Subsystem/nlsef/fal/If Action Subsystem  SystemSampleTime=-1  Latency=0  AutoFrameSizeCalculation=off
  Merge : Merge
  Product : Product
  Product1 : Product
  Sign : Signum
  Sum : Sum  Inputs=+-
  Sum1 : Sum  Inputs=|+-
  pow : Math  Operator=pow  SaturateOnIntegerOverflow=on
  pow1 : Math  Operator=pow  SaturateOnIntegerOverflow=on
  fal : Outport  VectorParamsAs1DForOutWhenUnconnected=off
  wires:
  d/1 -> Product1/1
  e/1 -> Abs/1, Divide/1, Sign/1  "x"
  Abs/1 -> Sum1/1, pow/1  "|x|"
  If Action Subsystem/1(Out1) -> Merge/2
  Sum1/1 -> If/1  "|x|-d"
  a/1 -> pow/2, Sum/2  "a"
  Product/1 -> If Action Subsystem2/1  "sign(x)|x|^a"
  Merge/1 -> fal/1
  Sum/1 -> pow1/2
  Product1/1 -> Sum1/2, pow1/1  "d"
  If/1 -> If Action Subsystem2/Action  "|x|>d"
  pow1/1 -> Divide/2  "d^(1-a)"
  Constant1/1 -> Sum/1, Product1/2
  If/2 -> If Action Subsystem/Action  "|x|<=d"
  pow/1 -> Product/2  "|x|^a"
  If Action Subsystem2/1 -> Merge/1
  Divide/1 -> If Action Subsystem/1(In1)
  Sign/1 -> Product/1  "sign(x)"

== system CopterSim3DEnvironment/ADRC_Controller /CSAS/angularRate_ADRC/ADRCController2/NLSEF/Subsystem/If Action Subsystem1 ==
  In1 : Inport
  Action Port : ActionPort
  Out1 : Outport
  wires:
  In1/1 -> Out1/1

== system CopterSim3DEnvironment/ADRC_Controller /CSAS/angularRate_ADRC/ADRCController2/NLSEF/Subsystem/If Action Subsystem3 ==
  In1 : Inport
  Action Port : ActionPort
  Out1 : Outport
  wires:
  In1/1 -> Out1/1

== system CopterSim3DEnvironment/ADRC_Controller /CSAS/angularRate_ADRC/ADRCController2/NLSEF/Subsystem1/If Action Subsystem1 ==
  In1 : Inport
  Action Port : ActionPort
  Out1 : Outport
  wires:
  In1/1 -> Out1/1

== system CopterSim3DEnvironment/ADRC_Controller /CSAS/angularRate_ADRC/ADRCController2/NLSEF/Subsystem1/If Action Subsystem3 ==
  In1 : Inport
  Action Port : ActionPort
  Out1 : Outport
  wires:
  In1/1 -> Out1/1

== system CopterSim3DEnvironment/ADRC_Controller /CSAS/angularRate_ADRC/ADRCController2/TD/fhan/Fhan ==
  a : Inport
  d : Inport  Port=2
  r : Inport  Port=3
  Abs : Abs
  If : If  NumInputs=2  IfExpression=u1 > u2
  If Action Subsystem : Subsystem  TreatAsAtomicUnit=on
  If Action Subsystem1 : Subsystem  TreatAsAtomicUnit=on
  Merge : Merge
  Out1 : Outport
  wires:
  a/1 -> If Action Subsystem1/2(a), If Action Subsystem/1(a), Abs/1
  d/1 -> If Action Subsystem1/3(d), If/2
  Abs/1 -> If/1
  If/1 -> If Action Subsystem/Action
  If/2 -> If Action Subsystem1/Action
  r/1 -> If Action Subsystem/2(r), If Action Subsystem1/1(r)
  If Action Subsystem/1(Out1) -> Merge/1
  If Action Subsystem1/1(Out1) -> Merge/2
  Merge/1 -> Out1/1

== system CopterSim3DEnvironment/ADRC_Controller /CSAS/angularRate_ADRC/ADRCController2/TD/fhan/a ==
  v2 : Inport
  a0 : Inport  Port=2
  d : Inport  Port=3
  y : Inport  Port=4
  d0 : Inport  Port=5
  h : Inport  Port=6
  Abs : Abs
  If : If  NumInputs=2  IfExpression=u1 > u2
  If Action Subsystem : Subsystem  TreatAsAtomicUnit=on
  If Action Subsystem1 : Subsystem  TreatAsAtomicUnit=on
  Merge : Merge
  a : Outport
  wires:
  v2/1 -> If Action Subsystem1/3(v2), If Action Subsystem/3(v2)
  y/1 -> If Action Subsystem/4(y), Abs/1, If Action Subsystem1/1(y)
  If/1 -> If Action Subsystem/Action
  If/2 -> If Action Subsystem1/Action
  Abs/1 -> If/1
  d0/1 -> If/2
  a0/1 -> If Action Subsystem/1(a0)
  d/1 -> If Action Subsystem/2(d)
  h/1 -> If Action Subsystem1/2(h)
  If Action Subsystem/1(Out2) -> Merge/1
  If Action Subsystem1/1(Out1) -> Merge/2
  Merge/1 -> a/1

== system CopterSim3DEnvironment/ADRC_Controller /CSAS/angularRate_ADRC/ADRCController2/TD/fhan/a0 ==
  d : Inport
  r : Inport  Port=2
  y : Inport  Port=3
  Abs : Abs
  Add : Sum
  Constant : Constant  Value=1/2
  Constant1 : Constant  Value=8
  Math Function : Math  Operator=pow  SignedPower=off  SaturateOnIntegerOverflow=on
  Math Function1 : Math  Operator=square  SignedPower=off  SaturateOnIntegerOverflow=on
  Product : Product  Inputs=3
  a0 : Outport
  wires:
  d/1 -> Math Function1/1
  Constant/1 -> Math Function/2
  Math Function1/1 -> Add/1
  r/1 -> Product/2
  Constant1/1 -> Product/1
  y/1 -> Abs/1
  Abs/1 -> Product/3
  Product/1 -> Add/2
  Add/1 -> Math Function/1
  Math Function/1 -> a0/1

== system CopterSim3DEnvironment/ADRC_Controller /CSAS/angularRate_ADRC/ADRCController2/TD/fhan/d ==
  r : Inport
  h : Inport  Port=2
  Product : Product
  d : Outport
  wires:
  r/1 -> Product/1
  h/1 -> Product/2
  Product/1 -> d/1

== system CopterSim3DEnvironment/ADRC_Controller /CSAS/angularRate_ADRC/ADRCController2/TD/fhan/d0 ==
  d : Inport
  h : Inport  Port=2
  Product : Product
  d0 : Outport
  wires:
  d/1 -> Product/1
  h/1 -> Product/2
  Product/1 -> d0/1

== system CopterSim3DEnvironment/ADRC_Controller /CSAS/angularRate_ADRC/ADRCController2/TD/fhan/y ==
  e : Inport
  v2 : Inport  Port=2
  h : Inport  Port=3
  Add : Sum
  Product : Product
  y : Outport
  wires:
  e/1 -> Add/1
  v2/1 -> Product/1
  h/1 -> Product/2
  Product/1 -> Add/2
  Add/1 -> y/1

== system CopterSim3DEnvironment/ADRC_Controller /CSAS/angularRate_ADRC/ADRCController2/eso/Subsystem/If Action Subsystem1 ==
  In1 : Inport
  Action Port : ActionPort
  Out1 : Outport
  wires:
  In1/1 -> Out1/1

== system CopterSim3DEnvironment/ADRC_Controller /CSAS/angularRate_ADRC/ADRCController2/eso/Subsystem/If Action Subsystem3 ==
  In1 : Inport
  Action Port : ActionPort
  Out1 : Outport
  wires:
  In1/1 -> Out1/1

== system CopterSim3DEnvironment/ADRC_Controller /CSAS/angularRate_ADRC/ADRCController2/eso/Subsystem1/If Action Subsystem ==
  In1 : Inport
  Action Port : ActionPort
  Out1 : Outport
  wires:
  In1/1 -> Out1/1

== system CopterSim3DEnvironment/ADRC_Controller /CSAS/angularRate_ADRC/ADRCController2/eso/Subsystem1/If Action Subsystem1 ==
  In1 : Inport
  Action Port : ActionPort
  Out1 : Outport
  wires:
  In1/1 -> Out1/1

== system CopterSim3DEnvironment/ADRC_Controller /CSAS/angularRate_ADRC/ADRCController3/Subsystem/nlsef/fal ==
  e : Inport
  a : Inport  Port=2
  d : Inport  Port=3
  Abs : Abs
  Constant1 : Constant  OutDataTypeStr=single
  Divide : Product  Inputs=*/
  If : If
  If Action Subsystem : Subsystem  TreatAsAtomicUnit=on
  If Action Subsystem2 : ctrl_ADRC_angular_rate/Subsystem/nlsef/fal/If Action Subsystem  SystemSampleTime=-1  Latency=0  AutoFrameSizeCalculation=off
  Merge : Merge
  Product : Product
  Product1 : Product
  Sign : Signum
  Sum : Sum  Inputs=+-
  Sum1 : Sum  Inputs=|+-
  pow : Math  Operator=pow  SaturateOnIntegerOverflow=on
  pow1 : Math  Operator=pow  SaturateOnIntegerOverflow=on
  fal : Outport  VectorParamsAs1DForOutWhenUnconnected=off
  wires:
  d/1 -> Product1/1
  e/1 -> Abs/1, Divide/1, Sign/1  "x"
  Abs/1 -> Sum1/1, pow/1  "|x|"
  If Action Subsystem/1(Out1) -> Merge/2
  Sum1/1 -> If/1  "|x|-d"
  a/1 -> pow/2, Sum/2  "a"
  Product/1 -> If Action Subsystem2/1  "sign(x)|x|^a"
  Merge/1 -> fal/1
  Sum/1 -> pow1/2
  Product1/1 -> Sum1/2, pow1/1  "d"
  If/1 -> If Action Subsystem2/Action  "|x|>d"
  pow1/1 -> Divide/2  "d^(1-a)"
  Constant1/1 -> Sum/1, Product1/2
  If/2 -> If Action Subsystem/Action  "|x|<=d"
  pow/1 -> Product/2  "|x|^a"
  If Action Subsystem2/1 -> Merge/1
  Divide/1 -> If Action Subsystem/1(In1)
  Sign/1 -> Product/1  "sign(x)"

== system CopterSim3DEnvironment/ADRC_Controller /CSAS/angularRate_ADRC/ADRCController1/Subsystem/nlsef/fal/If Action Subsystem ==
  In1 : Inport
  Action Port : ActionPort  ActionPortLabel=else
  Out1 : Outport  VectorParamsAs1DForOutWhenUnconnected=off
  wires:
  In1/1 -> Out1/1

== system CopterSim3DEnvironment/ADRC_Controller /CSAS/angularRate_ADRC/ADRCController2/TD/fhan/Fhan/If Action Subsystem ==
  a : Inport
  r : Inport  Port=2
  Action Port : ActionPort
  Product : Product
  Sign : Subsystem
  Out1 : Outport
  wires:
  a/1 -> Sign/1(In1)
  Sign/1(Out1) -> Product/1
  r/1 -> Product/2
  Product/1 -> Out1/1

== system CopterSim3DEnvironment/ADRC_Controller /CSAS/angularRate_ADRC/ADRCController2/TD/fhan/Fhan/If Action Subsystem1 ==
  r : Inport
  a : Inport  Port=2
  d : Inport  Port=3
  Action Port : ActionPort
  Divide : Product  Inputs=*/
  Product : Product
  Out1 : Outport
  wires:
  r/1 -> Product/1
  a/1 -> Divide/1
  d/1 -> Divide/2
  Divide/1 -> Product/2
  Product/1 -> Out1/1

== system CopterSim3DEnvironment/ADRC_Controller /CSAS/angularRate_ADRC/ADRCController2/TD/fhan/a/If Action Subsystem ==
  a0 : Inport
  d : Inport  Port=2
  v2 : Inport  Port=3
  y : Inport  Port=4
  Action Port : ActionPort
  Add : Sum  Inputs=-+
  Add1 : Sum
  Constant : Constant  Value=1/2
  Product : Product  Inputs=3
  Sign : Subsystem
  Out2 : Outport
  wires:
  Product/1 -> Add1/2
  Add/1 -> Product/1
  a0/1 -> Add/1
  d/1 -> Add/2
  Sign/1(Out1) -> Product/3
  Constant/1 -> Product/2
  Add1/1 -> Out2/1
  v2/1 -> Add1/1
  y/1 -> Sign/1(In1)

== system CopterSim3DEnvironment/ADRC_Controller /CSAS/angularRate_ADRC/ADRCController2/TD/fhan/a/If Action Subsystem1 ==
  y : Inport
  h : Inport  Port=2
  v2 : Inport  Port=3
  Action Port : ActionPort
  Add : Sum
  Divide : Product  Inputs=*/
  Out1 : Outport
  wires:
  y/1 -> Divide/1
  h/1 -> Divide/2
  v2/1 -> Add/2
  Divide/1 -> Add/1
  Add/1 -> Out1/1

== system CopterSim3DEnvironment/ADRC_Controller /CSAS/angularRate_ADRC/ADRCController3/Subsystem/nlsef/fal/If Action Subsystem ==
  In1 : Inport
  Action Port : ActionPort  ActionPortLabel=else
  Out1 : Outport  VectorParamsAs1DForOutWhenUnconnected=off
  wires:
  In1/1 -> Out1/1

== system CopterSim3DEnvironment/ADRC_Controller /CSAS/angularRate_ADRC/ADRCController2/TD/fhan/Fhan/If Action Subsystem/Sign ==
  In1 : Inport
  If : If  ElseIfExpressions=u1==0
  If Action Subsystem : Subsystem  TreatAsAtomicUnit=on
  If Action Subsystem1 : Subsystem  TreatAsAtomicUnit=on
  If Action Subsystem2 : Subsystem  TreatAsAtomicUnit=on
  Merge : Merge  Inputs=3
  Out1 : Outport
  wires:
  In1/1 -> If/1
  If/1 -> If Action Subsystem/Action
  If/2 -> If Action Subsystem1/Action
  If/3 -> If Action Subsystem2/Action
  If Action Subsystem/1(Out1) -> Merge/1
  If Action Subsystem1/1(Out1) -> Merge/2
  If Action Subsystem2/1(Out1) -> Merge/3
  Merge/1 -> Out1/1

== system CopterSim3DEnvironment/ADRC_Controller /CSAS/angularRate_ADRC/ADRCController2/TD/fhan/a/If Action Subsystem/Sign ==
  In1 : Inport
  If : If  ElseIfExpressions=u1==0
  If Action Subsystem : Subsystem  TreatAsAtomicUnit=on
  If Action Subsystem1 : Subsystem  TreatAsAtomicUnit=on
  If Action Subsystem2 : Subsystem  TreatAsAtomicUnit=on
  Merge : Merge  Inputs=3
  Out1 : Outport
  wires:
  In1/1 -> If/1
  If/1 -> If Action Subsystem/Action
  If/2 -> If Action Subsystem1/Action
  If/3 -> If Action Subsystem2/Action
  If Action Subsystem/1(Out1) -> Merge/1
  If Action Subsystem1/1(Out1) -> Merge/2
  If Action Subsystem2/1(Out1) -> Merge/3
  Merge/1 -> Out1/1

== system CopterSim3DEnvironment/ADRC_Controller /CSAS/angularRate_ADRC/ADRCController2/TD/fhan/Fhan/If Action Subsystem/Sign/If Action Subsystem ==
  Action Port : ActionPort
  Constant : Constant
  Out1 : Outport
  wires:
  Constant/1 -> Out1/1

== system CopterSim3DEnvironment/ADRC_Controller /CSAS/angularRate_ADRC/ADRCController2/TD/fhan/Fhan/If Action Subsystem/Sign/If Action Subsystem1 ==
  Action Port : ActionPort
  Constant : Constant  Value=0
  Out1 : Outport
  wires:
  Constant/1 -> Out1/1

== system CopterSim3DEnvironment/ADRC_Controller /CSAS/angularRate_ADRC/ADRCController2/TD/fhan/Fhan/If Action Subsystem/Sign/If Action Subsystem2 ==
  Action Port : ActionPort
  Constant : Constant  Value=-1
  Out1 : Outport
  wires:
  Constant/1 -> Out1/1

== system CopterSim3DEnvironment/ADRC_Controller /CSAS/angularRate_ADRC/ADRCController2/TD/fhan/a/If Action Subsystem/Sign/If Action Subsystem ==
  Action Port : ActionPort
  Constant : Constant
  Out1 : Outport
  wires:
  Constant/1 -> Out1/1

== system CopterSim3DEnvironment/ADRC_Controller /CSAS/angularRate_ADRC/ADRCController2/TD/fhan/a/If Action Subsystem/Sign/If Action Subsystem1 ==
  Action Port : ActionPort
  Constant : Constant  Value=0
  Out1 : Outport
  wires:
  Constant/1 -> Out1/1

== system CopterSim3DEnvironment/ADRC_Controller /CSAS/angularRate_ADRC/ADRCController2/TD/fhan/a/If Action Subsystem/Sign/If Action Subsystem2 ==
  Action Port : ActionPort
  Constant : Constant  Value=-1
  Out1 : Outport
  wires:
  Constant/1 -> Out1/1

== matlab function CopterSim3DEnvironment/Control System1/InputConditioning/MATLAB Function ==
  data: u input; y output
function y = fcn(u)
%将遥控输入的范围控制在1100~1900，同时设置一个死区，死区大小为±deadZone
RCMin = 1100;
RCMax = 1900;
deadZoneRate = 0.05;
deadZone = deadZoneRate*(RCMax-RCMin);
%限幅
if(u < RCMin)
    u = RCMin;
elseif(u > RCMax)
    u = RCMax;
end
%死区
 if(u > 1500+deadZone)
    y = u;
 elseif(u < 1500-deadZone)
     y = u;
 else
     y = 1500;
 end
     
 end

== matlab function CopterSim3DEnvironment/ADRC_Controller /InputConditioning/MATLAB Function ==
  data: u input; y output
function y = fcn(u)
%将遥控输入的范围控制在1100~1900，同时设置一个死区，死区大小为±deadZone
RCMin = 1100;
RCMax = 1900;
deadZoneRate = 0.05;
deadZone = deadZoneRate*(RCMax-RCMin);
%限幅
if(u < RCMin)
    u = RCMin;
elseif(u > RCMax)
    u = RCMax;
end
%死区
 if(u > 1500+deadZone)
    y = u;
 elseif(u < 1500-deadZone)
     y = u;
 else
     y = 1500;
 end
     
 end

== matlab function CopterSim3DEnvironment/ADRC_Controller /InputConditioning/MATLAB Function1 ==
  data: u input; y output
function y = fcn(u)
%将遥控输入的范围控制在1100~1900，同时设置一个死区，死区大小为±deadZone
RCMin = 1100;
RCMax = 1900;
deadZoneRate = 0.05;
deadZone = deadZoneRate*(RCMax-RCMin);
%限幅
if(u < RCMin)
    u = RCMin;
elseif(u > RCMax)
    u = RCMax;
end
%死区
 if(u > 1500+deadZone)
    y = u;
 elseif(u < 1500-deadZone)
     y = u;
 else
     y = 1500;
 end
     
 end

== matlab function CopterSim3DEnvironment/Control System1/InputConditioning/MATLAB Function1 ==
  data: u input; y output
function y = fcn(u)
%将遥控输入的范围控制在1100~1900，同时设置一个死区，死区大小为±deadZone
RCMin = 1100;
RCMax = 1900;
deadZoneRate = 0.05;
deadZone = deadZoneRate*(RCMax-RCMin);
%限幅
if(u < RCMin)
    u = RCMin;
elseif(u > RCMax)
    u = RCMax;
end
%死区
 if(u > 1500+deadZone)
    y = u;
 elseif(u < 1500-deadZone)
     y = u;
 else
     y = 1500;
 end
     
 end

== matlab function CopterSim3DEnvironment/ADRC_Controller /InputConditioning/MATLAB Function2 ==
  data: u input; y output
function y = fcn(u)
%将遥控输入的范围控制在1100~1900，同时设置一个死区，死区大小为±deadZone
RCMin = 1100;
RCMax = 1900;
deadZoneRate = 0.05;
deadZone = deadZoneRate*(RCMax-RCMin);
%限幅
if(u < RCMin)
    u = RCMin;
elseif(u > RCMax)
    u = RCMax;
end
%死区
 if(u > 1500+deadZone)
    y = u;
 elseif(u < 1500-deadZone)
     y = u;
 else
     y = 1500;
 end
     
 end

== matlab function CopterSim3DEnvironment/Control System1/InputConditioning/MATLAB Function2 ==
  data: u input; y output
function y = fcn(u)
%将遥控输入的范围控制在1100~1900，同时设置一个死区，死区大小为±deadZone
RCMin = 1100;
RCMax = 1900;
deadZoneRate = 0.05;
deadZone = deadZoneRate*(RCMax-RCMin);
%限幅
if(u < RCMin)
    u = RCMin;
elseif(u > RCMax)
    u = RCMax;
end
%死区
 if(u > 1500+deadZone)
    y = u;
 elseif(u < 1500-deadZone)
     y = u;
 else
     y = 1500;
 end
     
 end

== matlab function CopterSim3DEnvironment/ADRC_Controller /InputConditioning/MATLAB Function3 ==
  data: u input; y output
function y = fcn(u)
%将遥控输入的范围控制在1100~1900，同时设置一个死区，死区大小为±deadZone
RCMin = 1100;
RCMax = 1900;
deadZoneRate = 0.05;
deadZone = deadZoneRate*(RCMax-RCMin);
%限幅
if(u < RCMin)
    u = RCMin;
elseif(u > RCMax)
    u = RCMax;
end
%死区
 if(u > 1500+deadZone)
    y = u;
 elseif(u < 1500-deadZone)
     y = u;
 else
     y = 1500;
 end
     
 end

== matlab function CopterSim3DEnvironment/Control System1/pwm_out1 ==
  data: Roll input; M1 output; Pitch input; Yaw input; Thrust input; M2 output; M3 output; M4 output
function [M1, M2, M3, M4] = motor_mixer(Roll, Pitch, Yaw, Thrust)

idle_PWM = 1000;

% Quad XROLL （根据QP里面的叉字形结构的文字）
% M1 = ((Pitch+ Yaw)+Thrust-Roll) * 1000 + idle_PWM;
 %M2 = ((Pitch - Yaw)+Thrust+Roll) * 1000 + idle_PWM;
 %M3 = ((Roll +Yaw) + Thrust-Pitch) * 1000 + idle_PWM;
 %M4 = ((-Roll - Pitch-Yaw) + Thrust) * 1000 + idle_PWM;
% M5 = 1000;
% M6 = 1000;
% M7 = 1000;
% M8 = 1000;
%qp上实际的输出
M1 = (Thrust+Pitch-Roll+Yaw)*1000  + idle_PWM;
M2 = (Thrust-Pitch +Roll+Yaw)*1000 + idle_PWM;
M3 = (Thrust+Roll+Pitch-Yaw)*1000  + idle_PWM;
M4 = (Thrust-Roll- Pitch -Yaw)*1000 + idle_PWM;
% Quad +
 %M1 = ((Pitch - Yaw) * Thrust / 2 + Thrust) * 1000 + idle_PWM;
 %M2 = ((-Roll + Yaw) * Thrust / 2 + Thrust) * 1000 + idle_PWM;
% M3 = ((-Pitch - Yaw) * Thrust / 2 + Thrust) * 1000 + idle_PWM;
 %M4 = ((Roll + Yaw) * Thrust / 2 + Thrust) * 1000 + idle_PWM;
% M5 = 1000;
% M6 = 1000;
% M7 = 1000;
% M8 = 1000;

% Hex X
% M1 = ((Pitch + Roll / 2 - Yaw) * Thrust / 2 + Thrust) * 1000 + idle_PWM;
% M2 = ((Pitch - Roll / 2 + Yaw) * Thrust / 2 + Thrust) * 1000 + idle_PWM;
% M3 = ((-Roll - Yaw) * Thrust / 2 + Thrust) * 1000 + idle_PWM;
% M4 = ((-Pitch - Roll / 2 + Yaw) * Thrust / 2 + Thrust) * 1000 + idle_PWM;
% M5 = ((-Pitch + Roll / 2 - Yaw) * Thrust / 2 + Thrust) * 1000 + idle_PWM;
% M6 = ((Roll + Yaw) * Thrust / 2 + Thrust) * 1000 + idle_PWM;
% M7 = 1000;
% M8 = 1000;

% Hex X (From Adam)
%M1 = uint16(single(((-Roll - Yaw) * Thrust / 3 + Thrust) * single(1000))) + idle_PWM;
%M2 = uint16(single(((Roll + Yaw) * Thrust / 3 + Thrust) * single(1000))) + idle_PWM;
%M3 = uint16(single(((Pitch + (Roll / 2) - Yaw) * Thrust / 3 + Thrust) * single(1000))) + idle_PWM;
%M4 = uint16(single(((-Pitch - (Roll / 2) + Yaw) * Thrust / 3 + Thrust) * single(1000))) + idle_PWM;
%M5 = uint16(single(((Pitch - (Roll / 2) + Yaw) * Thrust / 3 + Thrust) * single(1000))) + idle_PWM;
%M6 = uint16(single(((-Pitch + (Roll / 2) - Yaw) * Thrust / 3 + Thrust) * single(1000))) + idle_PWM;

% Hex X (Version 2)
% Roll/Yaw
% M1 = ((-Roll - Yaw) * Thrust / 2 + Thrust) * 1000 + idle_PWM;
% M2 = ((Roll + Yaw) * Thrust / 2 + Thrust) * 1000 + idle_PWM;
% % + Pitch/Roll
% M6 = ((Pitch + Roll / 2 - Yaw) * Thrust / 2 + Thrust) * 1000 + idle_PWM;
% M4 = ((Pitch - Roll / 2 + Yaw) * Thrust / 2 + Thrust) * 1000 + idle_PWM;
% % - Pitch/Roll
% M5 = ((-Pitch - Roll / 2 + Yaw) * Thrust / 2 + Thrust) * 1000 + idle_PWM;
% M3 = ((-Pitch + Roll / 2 - Yaw) * Thrust / 2 + Thrust) * 1000 + idle_PWM;
